simulink library "control"  (R2024a)
settings: Solver=VariableStepAuto  StartTime=0.0  StopTime=10.0  RelTol=1e-3
libraries: vrlib x1
settings Model: Creator=leona  LastModifiedBy=leona

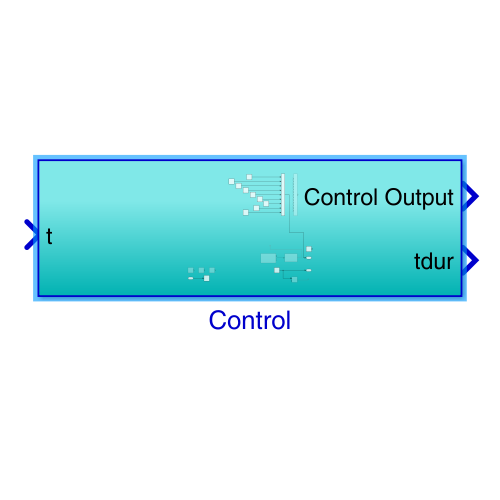
[thumbnail: Simulink's stored preview of the top-level diagram]
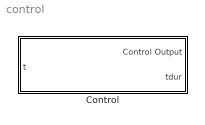
== system control ==
  Control : Subsystem

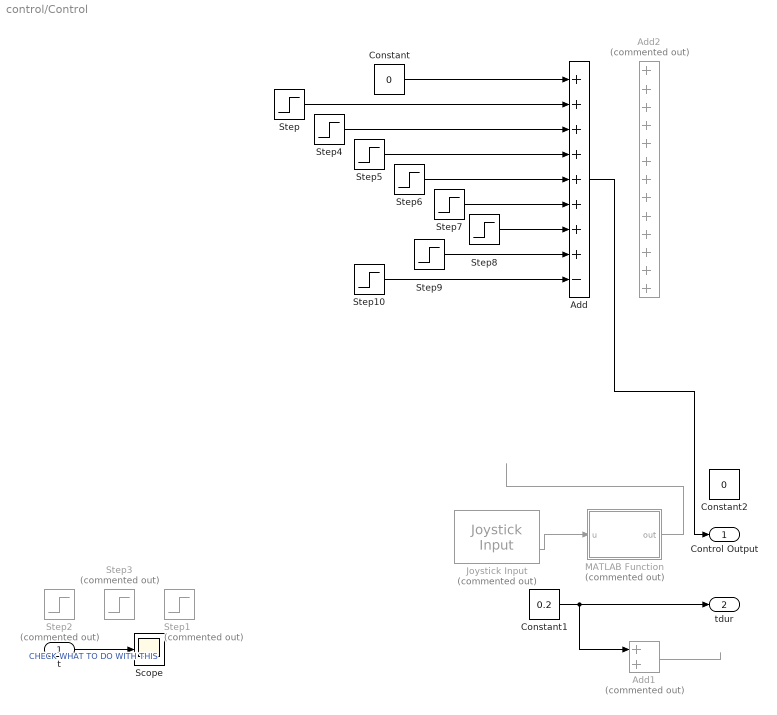
== system control/Control ==
  t : Inport
  Add : Sum  Inputs=++++++++-
  Add1 : Sum  Commented=on
  Add2 : Sum  Commented=on  Inputs=+++++++++++++
  Constant : Constant  Value=0
  Constant1 : Constant  Value=0.2
  Constant2 : Constant  Value=0
  Joystick Input : vrlib/Joystick Input  Commented=on  joyid=1  adjustports=on  forcefeed=off
  MATLAB Function : MATLAB Function  Commented=on  TreatAsAtomicUnit=on
  Scope : Scope
  Step : Step  After=2  SampleTime=0
  Step1 : Step  Commented=on  Time=3  After=-0.5  SampleTime=0
  Step10 : Step  Time=16  After=0  SampleTime=0
  Step2 : Step  Commented=on  After=2  SampleTime=0
  Step3 : Step  Commented=on  Time=0  Before=1  SampleTime=0
  Step4 : Step  Time=1.5  After=0  SampleTime=0
  Step5 : Step  Time=9  After=0  SampleTime=0
  Step6 : Step  Time=10  After=0  SampleTime=0
  Step7 : Step  Time=10  After=0  SampleTime=0
  Step8 : Step  Time=12  After=0  SampleTime=0
  Step9 : Step  Time=14  After=0  SampleTime=0
  Control Output : Outport
  tdur : Outport  Port=2
  wires:
  Step9/1 -> Add/8
  Step8/1 -> Add/7
  Step7/1 -> Add/6
  Step6/1 -> Add/5
  Step5/1 -> Add/4
  Step4/1 -> Add/3
  Step/1 -> Add/2
  Constant/1 -> Add/1
  Constant1/1 -> tdur/1, Add1/1
  Add1/1 -> ?
  t/1 -> Scope/1  "CHECK WHAT TO DO WITH THIS"
  Step10/1 -> Add/9
  Joystick Input/2 -> MATLAB Function/1(u)
  MATLAB Function/1(out) -> ?
  Add/1 -> Control Output/1

== matlab function control/Control/MATLAB Function ==
  data: u input; out output
function out = jsRead(u)

out = 0;
posVec = 0;

for i = 1:length(u)
    if u(i) == 1
        posVec = i;
    end
    
if posVec == 1 % walk backwards
    out = 3;
elseif posVec == 4 % walk forwards
    out = 1;
elseif posVec == 2 % walk right
    out = 5;
elseif posVec == 3 % walk left
    out = 4;
elseif posVec == 5 % turn left
    out = 6;
elseif posVec == 6 % turn right
    out = 7;
elseif posVec == 8 % trot
    out = 2;

end
end
